simulink model "thesismodel"  (R2018a)
settings: Solver=FixedStepAuto  StartTime=0.0  StopTime=15  FixedStep=0.01  RelTol=1e-3
undefined symbols (not defined in the file or in its folder): DiscIntNeverNeededParam, sigbuilder_block
libraries: simulink x3, dspstat3 x2
settings Model: Creator=qanta  LastModifiedBy=qanta

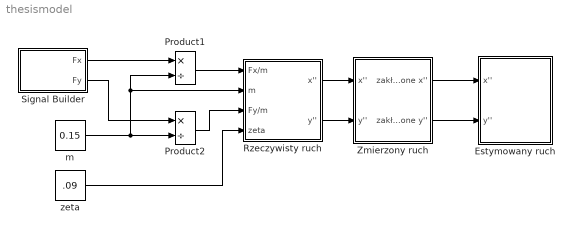
== system thesismodel ==
  Estymowany ruch : Subsystem
  Product1 : Product  Inputs=*/
  Product2 : Product  Inputs=*/
  Rzeczywisty ruch : Subsystem
  Signal Builder : Subsystem  Tag=STV Subsys  LoadFcn=sigbuilder_block('load');  StartFcn=sigbuilder_block('start');  StopFcn=sigbuilder_block('stop');  ClipboardFcn=sigbuilder_block('clipboard');  mask(Sigbuilder block){tuvar=[0:10]}
      mask help: Simulink:masks:SigbuilderBlock_MD
      mask init:
      | if ~strcmp(get_param(bdroot(gcbh),'SimulationStatus'),'stopped') tuvar = sigbuilder_block('maskInit'); end
      settings: CopyFcn=sigbuilder_block('copy');  DeleteFcn=sigbuilder_block('delete');  ModelCloseFcn=sigbuilder_block('modelClose');  PreSaveFcn=sigbuilder_block('preSave');  PauseFcn=sigbuilder_block('pause');  ContinueFcn=sigbuilder_block('continue');  NameChangeFcn=sigbuilder_block('namechange');  OpenFcn=sigbuilder_block('open',[75.5 61.5 550.5 362.5 ]);  CloseFcn=sigbuilder_block('close');
      mask Display: plot(0, 0, 100, 100,[2, 2, 32, 32, 2], [68, 8, 8, 68, 68],[32, 2], [38, 38], [32, 19, 2],[53, 60, 44], [32, 17, 17, 2],[16, 16, 31, 31]);txt = getActiveGroup(gcbh);text(2, 100, txt,'verticalAlignment', 'top');
  Zmierzony ruch : Subsystem
  m : Constant  Value=0.15
  zeta : Constant  Value=.09
  wires:
  Signal Builder/1(Fx) -> Product1/1
  m/1 -> Product1/2, Rzeczywisty ruch/2(m), Product2/2
  Signal Builder/2(Fy) -> Product2/1
  Product1/1 -> Rzeczywisty ruch/1(Fx/m)
  Product2/1 -> Rzeczywisty ruch/3(Fy/m)
  zeta/1 -> Rzeczywisty ruch/4(zeta)
  Rzeczywisty ruch/1(x'') -> Zmierzony ruch/1(x'')
  Rzeczywisty ruch/2(y'') -> Zmierzony ruch/2(y'')
  Zmierzony ruch/1(zakłócone x'') -> Estymowany ruch/1(x'')
  Zmierzony ruch/2(zakłócone y'') -> Estymowany ruch/2(y'')

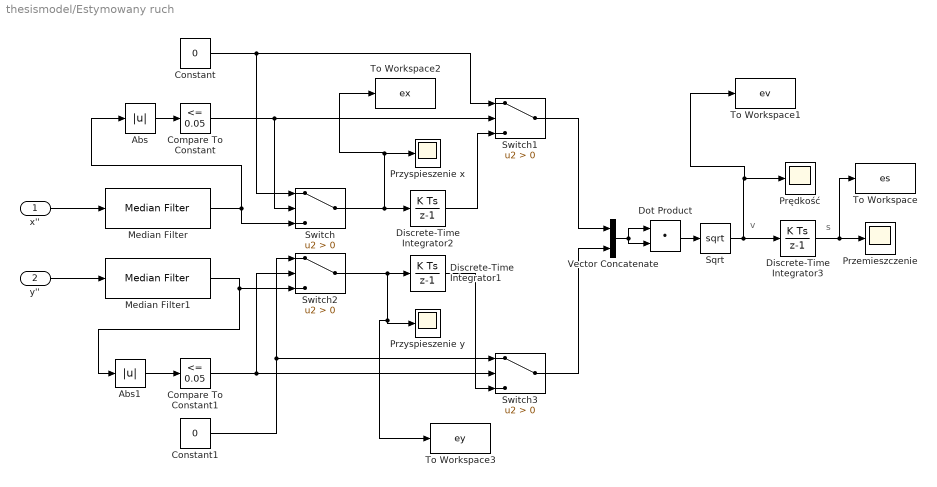
== system thesismodel/Estymowany ruch ==
  note: s
  note: v
  x'' : Inport
  y'' : Inport  Port=2
  Abs : Abs
  Abs1 : Abs
  Compare To Constant : simulink/Logic and Bit Operations/Compare To Constant  relop=<=  const=0.05  OutDataTypeStr=boolean
  Compare To Constant1 : simulink/Logic and Bit Operations/Compare To Constant  relop=<=  const=0.05  OutDataTypeStr=boolean
  Constant : Constant  Value=0
  Constant1 : Constant  Value=0
  Discrete-Time Integrator1 : DiscreteIntegrator  SampleTime=0.01  ICPrevOutput=DiscIntNeverNeededParam  ICPrevScaledInput=DiscIntNeverNeededParam
  Discrete-Time Integrator2 : DiscreteIntegrator  SampleTime=0.01  ICPrevOutput=DiscIntNeverNeededParam  ICPrevScaledInput=DiscIntNeverNeededParam
  Discrete-Time Integrator3 : DiscreteIntegrator  SampleTime=0.01  ICPrevOutput=DiscIntNeverNeededParam  ICPrevScaledInput=DiscIntNeverNeededParam
  Dot Product : DotProduct  InputSameDT=on  OutDataTypeStr=Inherit: Inherit via internal rule
  Median Filter : dspstat3/Median Filter  WindowLength=15  SimulateUsing=Interpreted execution
      settings: SourceProductName=DSP System Toolbox  SourceProductBaseCode=DS
  Median Filter1 : dspstat3/Median Filter  WindowLength=15  SimulateUsing=Interpreted execution
      settings: SourceProductName=DSP System Toolbox  SourceProductBaseCode=DS
  Przemieszczenie : Scope
  Przyspieszenie x : Scope
  Przyspieszenie y : Scope
  Prędkość : Scope
  Sqrt : Sqrt  SaturateOnIntegerOverflow=on
  Switch{,1..3} (4 alike) : Switch  Criteria=u2 > Threshold
  To Workspace : ToWorkspace  VariableName=es  SampleTime=-1
      settings: Save2DSignal=2-D array (concatenate along first dimension)
  To Workspace1 : ToWorkspace  VariableName=ev  SampleTime=-1
      settings: Save2DSignal=2-D array (concatenate along first dimension)
  To Workspace2 : ToWorkspace  VariableName=ex  SampleTime=-1
      settings: Save2DSignal=2-D array (concatenate along first dimension)
  To Workspace3 : ToWorkspace  VariableName=ey  SampleTime=-1
      settings: Save2DSignal=2-D array (concatenate along first dimension)
  Vector Concatenate : Concatenate
  wires:
  Discrete-Time Integrator3/1 -> To Workspace/1, Przemieszczenie/1
  Dot Product/1 -> Sqrt/1
  Vector Concatenate/1 -> Dot Product/1, Dot Product/2
  x''/1 -> Median Filter/1
  y''/1 -> Median Filter1/1
  Median Filter/1 -> Switch/3, Abs/1
  Compare To Constant/1 -> Switch/2, Switch1/2
  Switch/1 -> Discrete-Time Integrator2/1, To Workspace2/1, Przyspieszenie x/1
  Abs/1 -> Compare To Constant/1
  Constant/1 -> Switch1/1, Switch/1
  Constant1/1 -> Switch3/1, Switch2/1
  Compare To Constant1/1 -> Switch2/2, Switch3/2
  Median Filter1/1 -> Abs1/1, Switch2/3
  Switch2/1 -> To Workspace3/1, Przyspieszenie y/1, Discrete-Time Integrator1/1
  Sqrt/1 -> To Workspace1/1, Prędkość/1, Discrete-Time Integrator3/1
  Discrete-Time Integrator2/1 -> Switch1/3
  Switch1/1 -> Vector Concatenate/1
  Switch3/1 -> Vector Concatenate/2
  Discrete-Time Integrator1/1 -> Switch3/3
  Abs1/1 -> Compare To Constant1/1

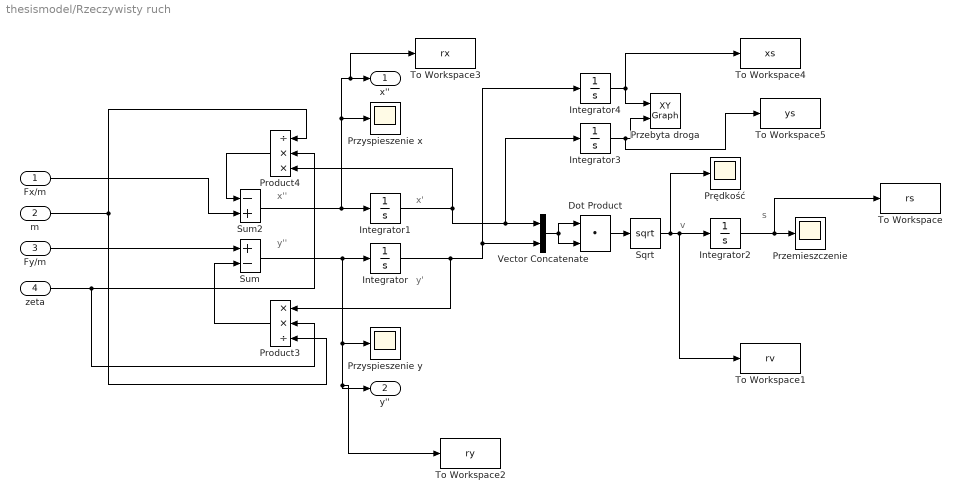
== system thesismodel/Rzeczywisty ruch ==
  note: s
  note: x'
  note: x''
  note: v
  note: y'
  note: y''
  Fx/m : Inport
  m : Inport  Port=2
  Fy/m : Inport  Port=3
  zeta : Inport  Port=4
  Dot Product : DotProduct  InputSameDT=on  OutDataTypeStr=Inherit: Inherit via internal rule
  Integrator{,1..4} (5 alike) : Integrator
  Product3 : Product  Inputs=**/
  Product4 : Product  Inputs=/**
  Przebyta droga : simulink/Sinks/XY Graph  xmin=-2.5  xmax=2.5  ymin=-2.5  ymax=2.5  st=-1
  Przemieszczenie : Scope
  Przyspieszenie x : Scope
  Przyspieszenie y : Scope
  Prędkość : Scope
  Sqrt : Sqrt  SaturateOnIntegerOverflow=on
  Sum : Sum  Inputs=+-
  Sum2 : Sum  Inputs=-+
  To Workspace : ToWorkspace  VariableName=rs  SaveFormat=Timeseries  SampleTime=-1
  To Workspace1 : ToWorkspace  VariableName=rv  SaveFormat=Timeseries  SampleTime=-1
  To Workspace2 : ToWorkspace  VariableName=ry  SaveFormat=Timeseries  SampleTime=-1
  To Workspace3 : ToWorkspace  VariableName=rx  SaveFormat=Timeseries  SampleTime=-1
  To Workspace4 : ToWorkspace  VariableName=xs  SampleTime=-1
      settings: Save2DSignal=2-D array (concatenate along first dimension)
  To Workspace5 : ToWorkspace  VariableName=ys  SampleTime=-1
      settings: Save2DSignal=2-D array (concatenate along first dimension)
  Vector Concatenate : Concatenate
  x'' : Outport
  y'' : Outport  Port=2
  wires:
  Integrator3/1 -> To Workspace5/1, Przebyta droga/2
  Integrator2/1 -> To Workspace/1, Przemieszczenie/1
  Integrator1/1 -> Integrator3/1, Vector Concatenate/1, Product4/3
  Integrator/1 -> Product3/1, Integrator4/1, Vector Concatenate/2
  Fy/m/1 -> Sum/1
  Sum/1 -> To Workspace2/1, y''/1, Przyspieszenie y/1, Integrator/1
  Sum2/1 -> Integrator1/1, To Workspace3/1, x''/1, Przyspieszenie x/1
  Product4/1 -> Sum2/1
  Sqrt/1 -> Prędkość/1, To Workspace1/1, Integrator2/1
  zeta/1 -> Product3/2, Product4/2
  Dot Product/1 -> Sqrt/1
  Vector Concatenate/1 -> Dot Product/1, Dot Product/2
  m/1 -> Product4/1, Product3/3
  Product3/1 -> Sum/2
  Integrator4/1 -> To Workspace4/1, Przebyta droga/1
  Fx/m/1 -> Sum2/2

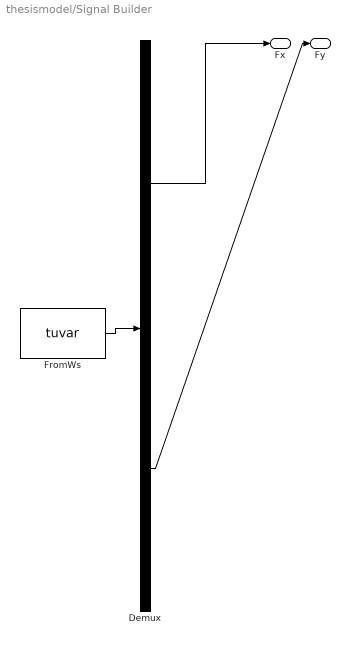
== system thesismodel/Signal Builder ==
  Demux : Demux  Tag=STV Demux  Outputs=2
  FromWs : FromWorkspace  Tag=STV FromWs  VariableName=tuvar  SampleTime=0
      SigBuilderData=|
      | common.afterFinalStr = 'Extrapolate'
      | common.sampleTime = 0
      | dataSet.timeRange = [0 10]
      | dataSet.name = 'Group 1'
      | sbobj.Groups.Name = 'Group 1'
      | sbobj.Groups.Signals(1).Name = 'Fx'
      | sbobj.Groups.Signals(1).XData = [0 1 1 10]
      | sbobj.Groups.Signals(1).YData = [0.2 0.2 0 0]
      | sbobj.Groups.Signals(2).Name = 'Fy'
      | sbobj.Groups.Signals(2).XData = [0 0.5 0.5 1.5 1.5 10]
      | sbobj.Groups.Signals(2).YData = [0 0 0.2 0.2 0 0]
  Fx : Outport  Tag=STV Outport
  Fy : Outport  Tag=STV Outport  Port=2
  wires:
  Demux/1 -> Fx/1
  FromWs/1 -> Demux/1
  Demux/2 -> Fy/1

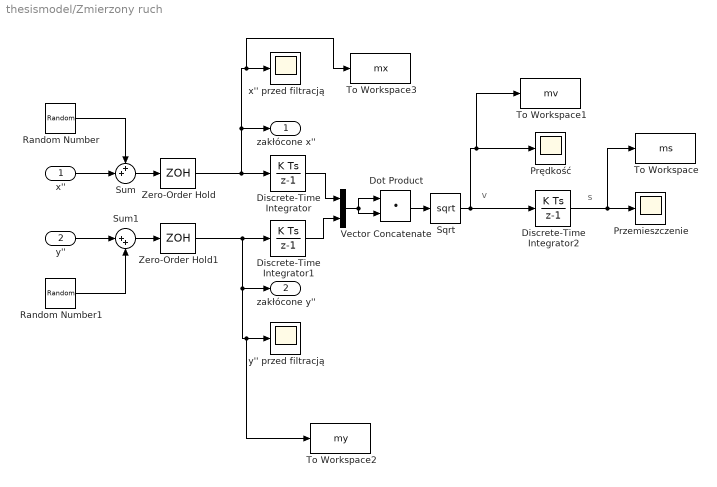
== system thesismodel/Zmierzony ruch ==
  note: s
  note: v
  x'' : Inport
  y'' : Inport  Port=2
  Discrete-Time Integrator : DiscreteIntegrator  SampleTime=0.01  ICPrevOutput=DiscIntNeverNeededParam  ICPrevScaledInput=DiscIntNeverNeededParam
  Discrete-Time Integrator1 : DiscreteIntegrator  SampleTime=0.01  ICPrevOutput=DiscIntNeverNeededParam  ICPrevScaledInput=DiscIntNeverNeededParam
  Discrete-Time Integrator2 : DiscreteIntegrator  SampleTime=0.01  ICPrevOutput=DiscIntNeverNeededParam  ICPrevScaledInput=DiscIntNeverNeededParam
  Dot Product : DotProduct  InputSameDT=on  OutDataTypeStr=Inherit: Inherit via internal rule
  Przemieszczenie : Scope
  Prędkość : Scope
  Random Number : RandomNumber  Mean=0.005  Variance=0.005  SampleTime=0.01
  Random Number1 : RandomNumber  Mean=0.005  Variance=0.005  SampleTime=0.01
  Sqrt : Sqrt  SaturateOnIntegerOverflow=on
  Sum : Sum  Inputs=++|
  Sum1 : Sum  Inputs=|++
  To Workspace : ToWorkspace  VariableName=ms  SaveFormat=Timeseries  SampleTime=-1
  To Workspace1 : ToWorkspace  VariableName=mv  SaveFormat=Timeseries  SampleTime=-1
  To Workspace2 : ToWorkspace  VariableName=my  SaveFormat=Timeseries  SampleTime=-1
  To Workspace3 : ToWorkspace  VariableName=mx  SaveFormat=Timeseries  SampleTime=-1
  Vector Concatenate : Concatenate
  Zero-Order Hold : ZeroOrderHold  SampleTime=0.01
  Zero-Order Hold1 : ZeroOrderHold  SampleTime=0.01
  x'' przed filtracją : Scope
  y'' przed filtracją : Scope
  zakłócone x'' : Outport
  zakłócone y'' : Outport  Port=2
  wires:
  Discrete-Time Integrator2/1 -> To Workspace/1, Przemieszczenie/1
  Sqrt/1 -> Discrete-Time Integrator2/1, To Workspace1/1, Prędkość/1
  Dot Product/1 -> Sqrt/1
  Vector Concatenate/1 -> Dot Product/1, Dot Product/2
  x''/1 -> Sum/2
  Random Number/1 -> Sum/1
  y''/1 -> Sum1/1
  Random Number1/1 -> Sum1/2
  Discrete-Time Integrator1/1 -> Vector Concatenate/2
  Discrete-Time Integrator/1 -> Vector Concatenate/1
  Sum/1 -> Zero-Order Hold/1
  Zero-Order Hold/1 -> Discrete-Time Integrator/1, zakłócone x''/1, To Workspace3/1, x'' przed filtracją/1
  Sum1/1 -> Zero-Order Hold1/1
  Zero-Order Hold1/1 -> Discrete-Time Integrator1/1, To Workspace2/1, y'' przed filtracją/1, zakłócone y''/1
